simulink model "fwd_and_inversekin"  (R2019a)
settings: Solver=VariableStepAuto  StartTime=0.0  StopTime=inf  RelTol=1e-3
libraries: mobileRoboticsLib x5
settings Model: Creator=xavifeds  LastModifiedBy=xavifeds

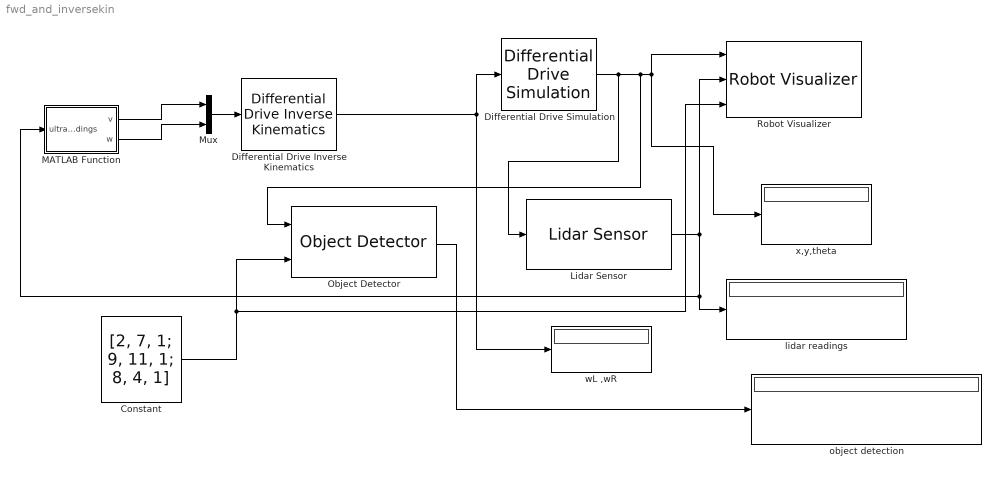
== system fwd_and_inversekin ==
  Constant : Constant  Value=[2, 7, 1; 9, 11, 1; 8, 4, 1]
  Differential Drive Inverse Kinematics : mobileRoboticsLib/Kinematic Models/Differential Drive/Differential Drive Inverse Kinematics  wheelRadius=0.04  wheelBase=0.13
      settings: SourceProductName=Mobile Robotics Simulation Toolbox
  Differential Drive Simulation : mobileRoboticsLib/Kinematic Models/Differential Drive/Differential Drive Simulation  wheelRadius=0.04  wheelBase=0.13  initX=1  initY=1  initAngle=pi/2  Ts=0.05
      settings: SourceProductName=Mobile Robotics Simulation Toolbox
  Lidar Sensor : mobileRoboticsLib/Environments/Lidar Sensor  mapName=map  sensorOffset=[ 0, 0 ]  scanAngles=[ -pi/2,0,pi/2]  maxRange=20
      settings: SourceProductName=Mobile Robotics Simulation Toolbox
  MATLAB Function : MATLAB Function  TreatAsAtomicUnit=on
  Mux : Mux  Inputs=2
  Object Detector : mobileRoboticsLib/Environments/Object Detector  sensorOffset=[ 0, 0 ]  sensorAngle=0  fieldOfView=pi/3  maxRange=5  maxDetections=3  sampleTime=0.1
      settings: SourceProductName=Mobile Robotics Simulation Toolbox
  Robot Visualizer : mobileRoboticsLib/Environments/Robot Visualizer  robotRadius=0  mapName=map  showTrajectory=on  hasWaypoints=off  hasLidar=on  sensorOffset=[ 0, 0 ]  scanAngles=[ -pi/2,0,pi/2]  hasObjDetector=on  objDetectorOffset=[ 0, 0 ]  objDetectorAngle=0  objDetectorFOV=pi/4  objDetectorMaxRange=5  objectColors=[ 1, 0, 0; 0, 1, 0; 0, 0, 1 ]  objectMarkers=s
  lidar readings : Display
  object detection : Display
  wL ,wR : Display
  x,y,theta : Display
  wires:
  Differential Drive Inverse Kinematics/1 -> wL ,wR/1, Differential Drive Simulation/1
  Differential Drive Simulation/1 -> Lidar Sensor/1, Object Detector/1, x,y,theta/1, Robot Visualizer/1
  Lidar Sensor/1 -> MATLAB Function/1(ultrasonic_readings), lidar readings/1, Robot Visualizer/2
  MATLAB Function/1(v) -> Mux/1
  MATLAB Function/2(w) -> Mux/2
  Mux/1 -> Differential Drive Inverse Kinematics/1
  Constant/1 -> Robot Visualizer/3, Object Detector/2
  Object Detector/1 -> object detection/1

== matlab function fwd_and_inversekin/MATLAB Function ==
  data: ultrasonic_readings input; v output; w output
function [v,w] = fcn(ultrasonic_readings)
dl = ultrasonic_readings(3);
df = ultrasonic_readings(2);
dr = ultrasonic_readings(1);
d = 1;
    if df > d && dl > d && dr > d
        [v,w] = change_state(0);
    elseif df < d && dl > d && dr > d
        [v,w] = change_state(1);
    elseif df > d && dl > d && dr < d
        [v,w] = change_state(2);
    elseif df > d && dl < d && dr > d
        [v,w] = change_state(0);
    elseif df < d && dl > d && dr < d
        [v,w] = change_state(1);
    elseif df < d && dl < d && dr > d
        [v,w] = change_state(1);
    elseif df < d && dl < d && dr < d
        [v,w] = change_state(1);
    elseif df > d && dl < d && dr < d
        [v,w] = change_state(0);
    else
        [v,w] = change_state(3);
    end
end

function [v,w] = change_state(value)
    if value == 0 
        v = 0.2;
        w = -0.3;
    end
    if value == 1 %turn lefft
        v = 0;
        w = 0.3;
        
    end
    if value == 2
        v = 0.5;
        w = 0;
    end
    if value == 3
        v = 0.2;
        w = -0.3;
    end
end
